simulink library "state_manager_lib"  (R2016b)
settings: Solver=ode45  StartTime=0.0  StopTime=10.0  RelTol=1e-3  EnableMultiTasking=on
undefined symbols (not defined in the file): ase_imu_p_indx, ase_local_mode_docking, ase_local_mode_map, ase_local_mode_perching, ase_ml_p_indx, ase_of_num_aug, ase_of_p_indx, ase_total_num_states, aug_state_enum, ml_omega_aug, ml_P_cam_ISS_ISS, ml_quat_ISS2cam, ml_vel_aug, of_omega_aug, of_vel_aug, tun_abp_p_dockcam_imu_est, tun_abp_p_navcam_imu_est, tun_abp_p_perchcam_imu_est, tun_abp_q_body2dockcam, tun_abp_q_body2navcam, tun_abp_q_body2perchcam, tun_ase_enable_of, tun_ase_ml_forward_projection_time
libraries: math_utils x8, simulink x7
settings Model: Creator=jfusco1  LastModifiedBy=jfusco1
settings DataIOCC: LimitDataPoints=on  SaveFormat=Array
settings OptimizationCC: LifeSpan=inf
settings DebuggingCC: AllowSymbolicDim=off  SFUnexpectedBacktrackingDiag=warning  SFNoUnconditionalDefaultTransitionDiag=warning  SFExecutionAtInitializationDiag=none
settings HardwareCC: ProdBitPerPointer=32  ProdBitPerSizeT=32  ProdBitPerPtrDiffT=32  ProdLargestAtomicFloat=None  ProdIntDivRoundTo=Undefined  ProdEndianess=Unspecified  ProdWordSize=32  ProdHWDeviceType=32-bit Generic
settings ModelReferenceCC: PropagateSignalLabelsOutOfModel=off
settings GRTTargetCC: TargetLangStandard=C89/C90 (ANSI)  GeneratePreprocessorConditionals=Disable all
settings ConfigComp: CovMetricSettings=dw  CovHtmlReporting=on  CovSaveCumulativeToWorkspaceVar=on  CovSaveSingleToWorkspaceVar=on  CovExternalEMLEnable=off

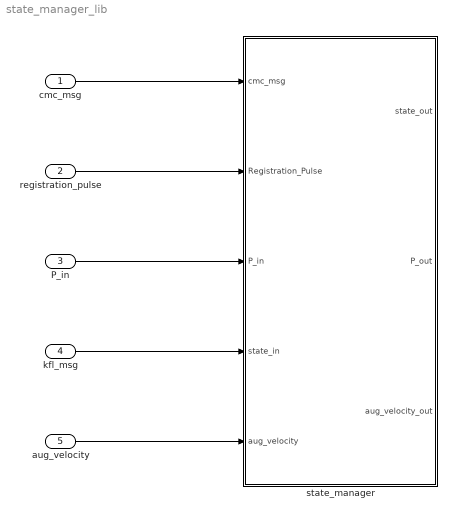
== system state_manager_lib ==
  cmc_msg : Inport  OutDataTypeStr=Bus: cmc_msg
  registration_pulse : Inport  Port=2  OutDataTypeStr=Bus: cvs_registration_pulse
  P_in : Inport  Port=3
  kfl_msg : Inport  Port=4  OutDataTypeStr=Bus: kfl_msg
  aug_velocity : Inport  Port=5
  state_manager : Subsystem
  wires:
  registration_pulse/1 -> state_manager/2(Registration_Pulse)
  kfl_msg/1 -> state_manager/4(state_in)
  P_in/1 -> state_manager/3(P_in)
  aug_velocity/1 -> state_manager/5(aug_velocity)
  cmc_msg/1 -> state_manager/1(cmc_msg)

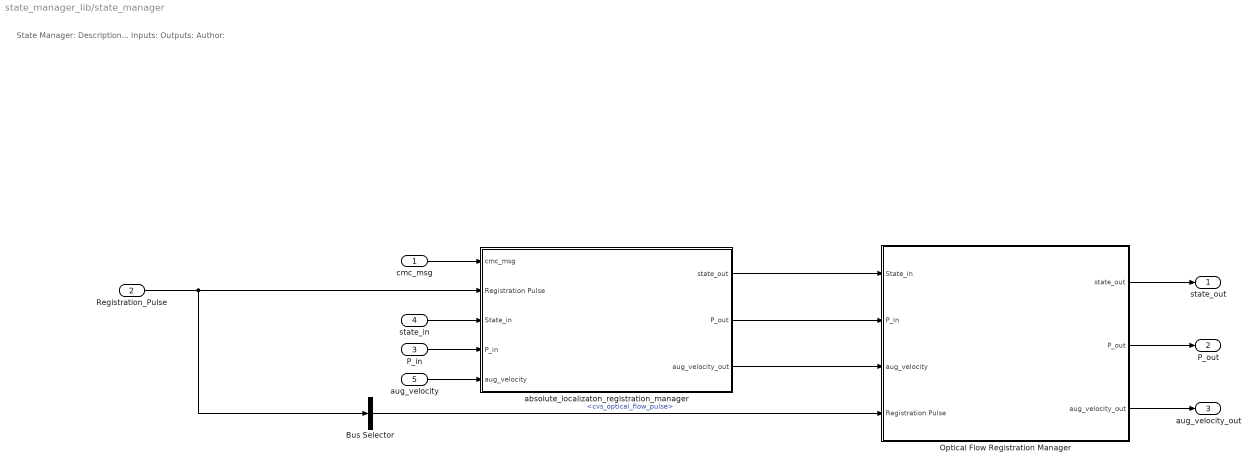
== system state_manager_lib/state_manager ==
  note: State Manager:
      | Description...
      |
      | Inputs:
      |
      | Outputs:
      |
      | Author:
  cmc_msg : Inport
  Registration_Pulse : Inport  Port=2
  P_in : Inport  Port=3  OutDataTypeStr=ase_cov_datatype
  state_in : Inport  Port=4
  aug_velocity : Inport  Port=5
  Bus Selector : BusSelector  OutputSignals=cvs_optical_flow_pulse
  Optical Flow Registration Manager : Subsystem
  absolute_localizaton_registration_manager : Subsystem
  state_out : Outport
  P_out : Outport  Port=2
  aug_velocity_out : Outport  Port=3
  wires:
  Optical Flow Registration Manager/3(aug_velocity_out) -> aug_velocity_out/1
  absolute_localizaton_registration_manager/3(aug_velocity_out) -> Optical Flow Registration Manager/3(aug_velocity)
  aug_velocity/1 -> absolute_localizaton_registration_manager/5(aug_velocity)
  state_in/1 -> absolute_localizaton_registration_manager/3(State_in)
  P_in/1 -> absolute_localizaton_registration_manager/4(P_in)
  absolute_localizaton_registration_manager/1(state_out) -> Optical Flow Registration Manager/1(State_in)
  Registration_Pulse/1 -> Bus Selector/1, absolute_localizaton_registration_manager/2(Registration Pulse)
  Bus Selector/1 -> Optical Flow Registration Manager/4(Registration Pulse)  "<cvs_optical_flow_pulse>"
  Optical Flow Registration Manager/1(state_out) -> state_out/1
  Optical Flow Registration Manager/2(P_out) -> P_out/1
  absolute_localizaton_registration_manager/2(P_out) -> Optical Flow Registration Manager/2(P_in)
  cmc_msg/1 -> absolute_localizaton_registration_manager/1(cmc_msg)

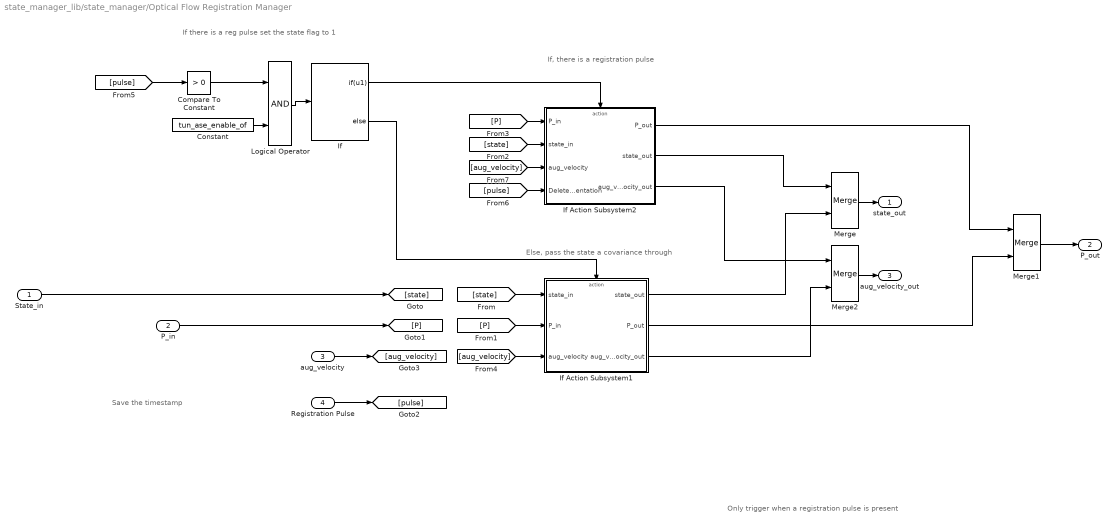
== system state_manager_lib/state_manager/Optical Flow Registration Manager ==
  note: Only trigger when a registration pulse is present
  note: If, there is a registration pulse
  note: Else, pass the state a covariance through
  note: Save the timestamp
  note: If there is a reg pulse set the state flag to 1
  State_in : Inport
  P_in : Inport  Port=2
  aug_velocity : Inport  Port=3
  Registration Pulse : Inport  Port=4
  Compare To Constant : simulink/Logic and Bit Operations/Compare To Constant  relop=>  const=0  OutDataTypeStr=boolean
  Constant : Constant  Value=tun_ase_enable_of
  If : If  IfExpression=u1
  If Action Subsystem1 : Subsystem  TreatAsAtomicUnit=on
  If Action Subsystem2 : Subsystem  TreatAsAtomicUnit=on
  Logical Operator : Logic  AllPortsSameDT=off  OutDataTypeStr=boolean
  Merge : Merge
  Merge1 : Merge
  Merge2 : Merge
  state_out : Outport
  P_out : Outport  Port=2
  aug_velocity_out : Outport  Port=3
  wires:
  If Action Subsystem1/3(aug_velocity_out) -> Merge2/2
  If Action Subsystem2/3(aug_velocity_out) -> Merge2/1
  Merge2/1 -> aug_velocity_out/1
  [aug_velocity] -> If Action Subsystem1/3(aug_velocity)
  [aug_velocity] -> If Action Subsystem2/3(aug_velocity)
  aug_velocity/1 -> [aug_velocity]
  [state] -> If Action Subsystem1/1(state_in)
  P_in/1 -> [P]
  [P] -> If Action Subsystem1/2(P_in)
  If/2 -> If Action Subsystem1/Action
  If/1 -> If Action Subsystem2/Action
  If Action Subsystem2/2(state_out) -> Merge/1
  [state] -> If Action Subsystem2/2(state_in)
  [P] -> If Action Subsystem2/1(P_in)
  If Action Subsystem2/1(P_out) -> Merge1/1
  Merge/1 -> state_out/1
  Merge1/1 -> P_out/1
  Logical Operator/1 -> If/1
  Compare To Constant/1 -> Logical Operator/1
  Constant/1 -> Logical Operator/2
  If Action Subsystem1/1(state_out) -> Merge/2
  If Action Subsystem1/2(P_out) -> Merge1/2
  State_in/1 -> [state]
  Registration Pulse/1 -> [pulse]
  [pulse] -> Compare To Constant/1
  [pulse] -> If Action Subsystem2/4(Deleted Augmentation)

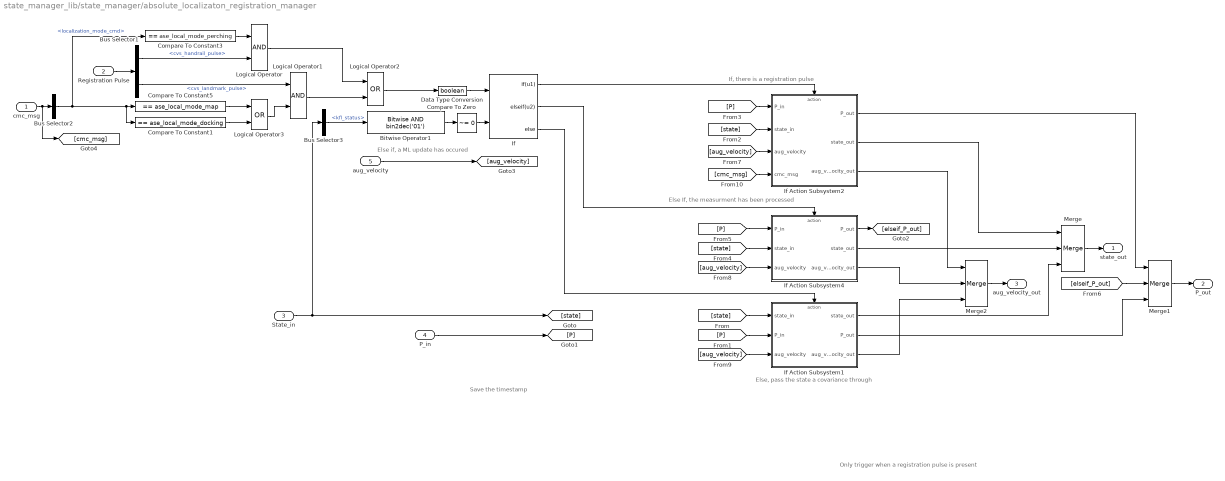
== system state_manager_lib/state_manager/absolute_localizaton_registration_manager ==
  note: Else If, the measurment has been processed
  note: Save the timestamp
  note: Else, pass the state a covariance through
  note: If, there is a registration pulse
  note: Only trigger when a registration pulse is present
  note: Else if, a ML update has occured
  cmc_msg : Inport
  Registration Pulse : Inport  Port=2
  State_in : Inport  Port=3
  P_in : Inport  Port=4
  aug_velocity : Inport  Port=5
  Bitwise Operator1 : simulink/Logic and Bit Operations/Bitwise Operator  logicop=AND  UseBitMask=on  BitMask=bin2dec('01')  BitMaskRealWorld=Stored Integer
  Bus Selector1 : BusSelector  OutputSignals=cvs_handrail_pulse,cvs_landmark_pulse
  Bus Selector2 : BusSelector  OutputSignals=localization_mode_cmd
  Bus Selector3 : BusSelector  OutputSignals=kfl_status
  Compare To Constant1 : simulink/Logic and Bit Operations/Compare To Constant  relop===  const=ase_local_mode_docking  OutDataTypeStr=boolean
  Compare To Constant3 : simulink/Logic and Bit Operations/Compare To Constant  relop===  const=ase_local_mode_perching  OutDataTypeStr=boolean
  Compare To Constant5 : simulink/Logic and Bit Operations/Compare To Constant  relop===  const=ase_local_mode_map  OutDataTypeStr=boolean
  Compare To Zero : simulink/Logic and Bit Operations/Compare To Zero  relop=~=  OutDataTypeStr=boolean
  Data Type Conversion : DataTypeConversion  OutDataTypeStr=boolean
  If : If  NumInputs=2  IfExpression=u1  ElseIfExpressions=u2
  If Action Subsystem1 : Subsystem  TreatAsAtomicUnit=on
  If Action Subsystem2 : Subsystem  TreatAsAtomicUnit=on
  If Action Subsystem4 : Subsystem  TreatAsAtomicUnit=on
  Logical Operator : Logic  AllPortsSameDT=off  OutDataTypeStr=boolean
  Logical Operator1 : Logic  AllPortsSameDT=off  OutDataTypeStr=boolean
  Logical Operator2 : Logic  Operator=OR  AllPortsSameDT=off  OutDataTypeStr=boolean
  Logical Operator3 : Logic  Operator=OR  AllPortsSameDT=off  OutDataTypeStr=boolean
  Merge : Merge  Inputs=3
  Merge1 : Merge  Inputs=3
  Merge2 : Merge  Inputs=3
  state_out : Outport
  P_out : Outport  Port=2
  aug_velocity_out : Outport  Port=3
  wires:
  If Action Subsystem1/3(aug_velocity_out) -> Merge2/3
  If Action Subsystem4/3(aug_velocity_out) -> Merge2/2
  If Action Subsystem2/3(aug_velocity_out) -> Merge2/1
  Merge2/1 -> aug_velocity_out/1
  [aug_velocity] -> If Action Subsystem1/3(aug_velocity)
  [aug_velocity] -> If Action Subsystem4/3(aug_velocity)
  [aug_velocity] -> If Action Subsystem2/3(aug_velocity)
  aug_velocity/1 -> [aug_velocity]
  Merge1/1 -> P_out/1
  [P] -> If Action Subsystem4/1(P_in)
  [state] -> If Action Subsystem4/2(state_in)
  Merge/1 -> state_out/1
  If Action Subsystem2/1(P_out) -> Merge1/1
  [P] -> If Action Subsystem2/1(P_in)
  If/2 -> If Action Subsystem4/Action
  [state] -> If Action Subsystem2/2(state_in)
  If Action Subsystem2/2(state_out) -> Merge/1
  If/1 -> If Action Subsystem2/Action
  If/3 -> If Action Subsystem1/Action
  [P] -> If Action Subsystem1/2(P_in)
  P_in/1 -> [P]
  [state] -> If Action Subsystem1/1(state_in)
  If Action Subsystem1/2(P_out) -> Merge1/3
  [elseif_P_out] -> Merge1/2
  Data Type Conversion/1 -> If/1
  If Action Subsystem4/1(P_out) -> [elseif_P_out]
  If Action Subsystem1/1(state_out) -> Merge/3
  If Action Subsystem4/2(state_out) -> Merge/2
  State_in/1 -> [state], Bus Selector3/1
  Bus Selector3/1 -> Bitwise Operator1/1  "<kfl_status>"
  Compare To Zero/1 -> If/2
  Bitwise Operator1/1 -> Compare To Zero/1
  Bus Selector2/1 -> Compare To Constant3/1, Compare To Constant1/1, Compare To Constant5/1  "<localization_mode_cmd>"
  cmc_msg/1 -> [cmc_msg], Bus Selector2/1
  Registration Pulse/1 -> Bus Selector1/1
  Logical Operator2/1 -> Data Type Conversion/1
  Logical Operator1/1 -> Logical Operator2/2
  Logical Operator/1 -> Logical Operator2/1
  Bus Selector1/1 -> Logical Operator/2  "<cvs_handrail_pulse>"
  Bus Selector1/2 -> Logical Operator1/1  "<cvs_landmark_pulse>"
  Compare To Constant3/1 -> Logical Operator/1
  [cmc_msg] -> If Action Subsystem2/4(cmc_msg)
  Compare To Constant5/1 -> Logical Operator3/1
  Compare To Constant1/1 -> Logical Operator3/2
  Logical Operator3/1 -> Logical Operator1/2

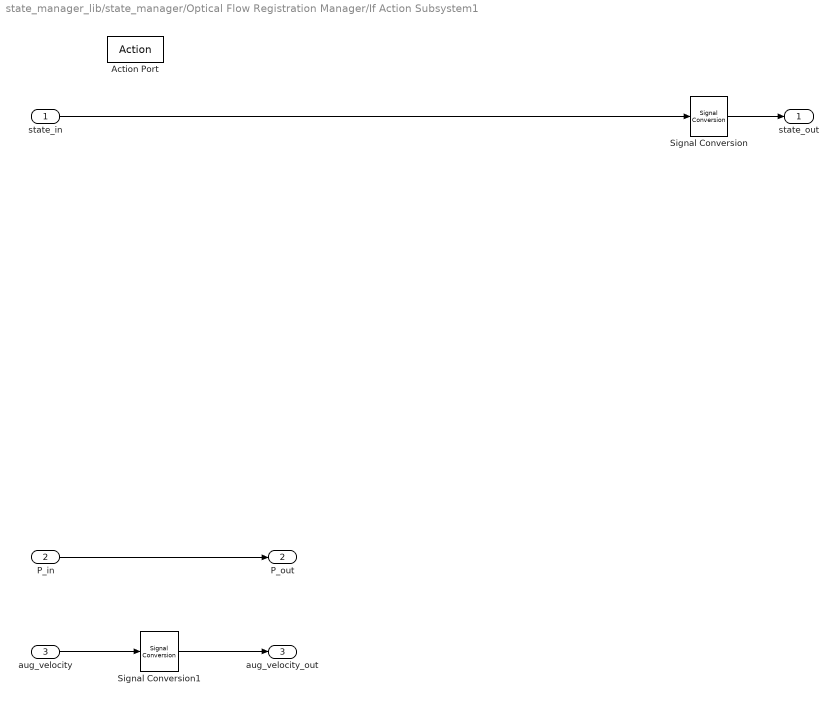
== system state_manager_lib/state_manager/Optical Flow Registration Manager/If Action Subsystem1 ==
  state_in : Inport
  P_in : Inport  Port=2
  aug_velocity : Inport  Port=3
  Action Port : ActionPort
  Signal Conversion : SignalConversion  OverrideOpt=off
  Signal Conversion1 : SignalConversion  OverrideOpt=off
  state_out : Outport
  P_out : Outport  Port=2
  aug_velocity_out : Outport  Port=3
  wires:
  Signal Conversion1/1 -> aug_velocity_out/1
  aug_velocity/1 -> Signal Conversion1/1
  P_in/1 -> P_out/1
  Signal Conversion/1 -> state_out/1
  state_in/1 -> Signal Conversion/1

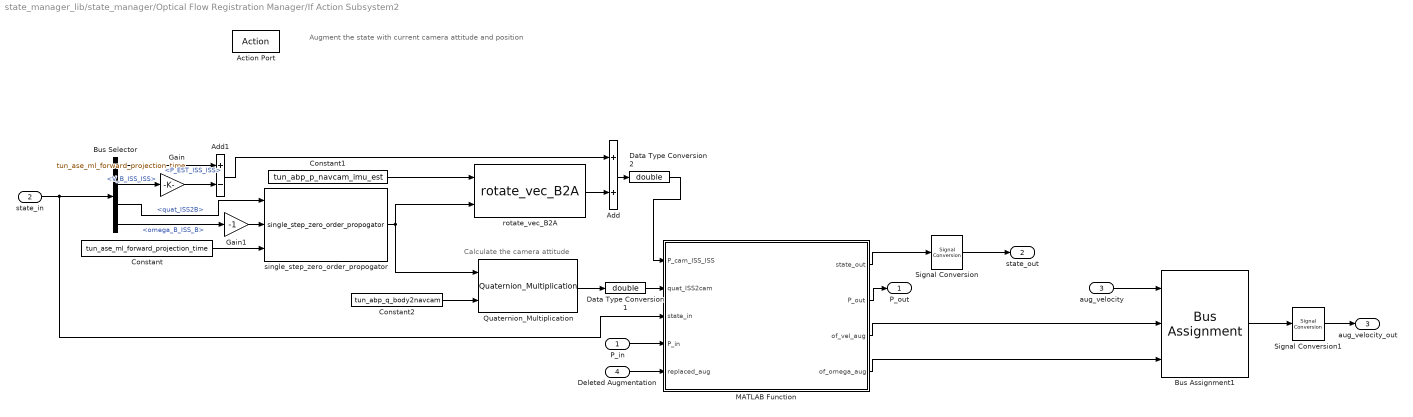
== system state_manager_lib/state_manager/Optical Flow Registration Manager/If Action Subsystem2 ==
  note: Augment the state with current camera attitude and position
  note: Calculate the camera attitude
  P_in : Inport
  state_in : Inport  Port=2
  aug_velocity : Inport  Port=3
  Deleted Augmentation : Inport  Port=4
  Action Port : ActionPort
  Add : Sum
  Add1 : Sum  Inputs=+-
  Bus Assignment1 : BusAssignment  AssignedSignals=of_vel_aug,of_omega_aug
  Bus Selector : BusSelector  OutputSignals=P_EST_ISS_ISS,V_B_ISS_ISS,quat_ISS2B,omega_B_ISS_B
  Constant : Constant  Value=tun_ase_ml_forward_projection_time
  Constant1 : Constant  Value=tun_abp_p_navcam_imu_est
  Constant2 : Constant  Value=tun_abp_q_body2navcam
  Data Type Conversion1 : DataTypeConversion  OutDataTypeStr=double
  Data Type Conversion2 : DataTypeConversion  OutDataTypeStr=double
  Gain : Gain  Gain=tun_ase_ml_forward_projection_time
  Gain1 : Gain  Gain=-1
  MATLAB Function : MATLAB Function  TreatAsAtomicUnit=on
  Quaternion_Multiplication : math_utils/Quaternion_Multiplication  SystemSampleTime=-1
  Signal Conversion : SignalConversion  OverrideOpt=off
  Signal Conversion1 : SignalConversion  OverrideOpt=off
  rotate_vec_B2A : math_utils/rotate_vec_B2A  SystemSampleTime=-1
  single_step_zero_order_propogator : math_utils/single_step_zero_order_propogator  SystemSampleTime=-1
  P_out : Outport
  state_out : Outport  Port=2
  aug_velocity_out : Outport  Port=3
  wires:
  Signal Conversion1/1 -> aug_velocity_out/1
  Bus Assignment1/1 -> Signal Conversion1/1
  MATLAB Function/4(of_omega_aug) -> Bus Assignment1/3
  MATLAB Function/3(of_vel_aug) -> Bus Assignment1/2
  aug_velocity/1 -> Bus Assignment1/1
  MATLAB Function/1(state_out) -> Signal Conversion/1
  state_in/1 -> MATLAB Function/3(state_in), Bus Selector/1
  Constant2/1 -> Quaternion_Multiplication/2
  Bus Selector/3 -> single_step_zero_order_propogator/1  "<quat_ISS2B>"
  Quaternion_Multiplication/1 -> Data Type Conversion1/1
  P_in/1 -> MATLAB Function/4(P_in)
  MATLAB Function/2(P_out) -> P_out/1
  Signal Conversion/1 -> state_out/1
  Bus Selector/4 -> Gain1/1  "<omega_B_ISS_B>"
  Gain1/1 -> single_step_zero_order_propogator/2
  Constant/1 -> single_step_zero_order_propogator/3
  Gain/1 -> Add1/2
  Add1/1 -> Add/1
  rotate_vec_B2A/1 -> Add/2
  Bus Selector/2 -> Gain/1  "<V_B_ISS_ISS>"
  Bus Selector/1 -> Add1/1  "<P_EST_ISS_ISS>"
  Constant1/1 -> rotate_vec_B2A/1
  Data Type Conversion1/1 -> MATLAB Function/2(quat_ISS2cam)
  Data Type Conversion2/1 -> MATLAB Function/1(P_cam_ISS_ISS)
  Add/1 -> Data Type Conversion2/1
  Deleted Augmentation/1 -> MATLAB Function/5(replaced_aug)
  single_step_zero_order_propogator/1 -> Quaternion_Multiplication/1, rotate_vec_B2A/2

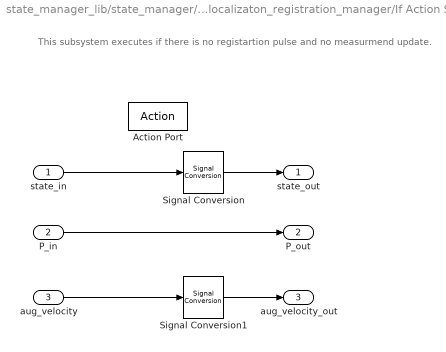
== system state_manager_lib/state_manager/absolute_localizaton_registration_manager/If Action Subsystem1 ==
  note: This subsystem executes if there is no registartion pulse and no measurmend update.
  state_in : Inport
  P_in : Inport  Port=2
  aug_velocity : Inport  Port=3
  Action Port : ActionPort
  Signal Conversion : SignalConversion  OverrideOpt=off
  Signal Conversion1 : SignalConversion  OverrideOpt=off
  state_out : Outport
  P_out : Outport  Port=2
  aug_velocity_out : Outport  Port=3
  wires:
  Signal Conversion1/1 -> aug_velocity_out/1
  aug_velocity/1 -> Signal Conversion1/1
  Signal Conversion/1 -> state_out/1
  P_in/1 -> P_out/1
  state_in/1 -> Signal Conversion/1

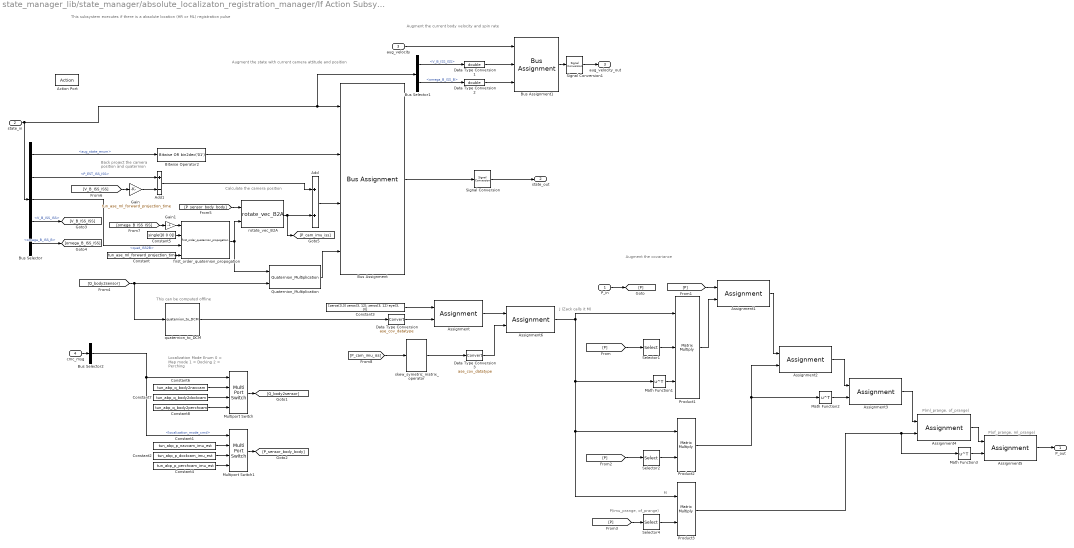
== system state_manager_lib/state_manager/absolute_localizaton_registration_manager/If Action Subsystem2 ==
  note: This subsystem executes if there is a absolute location (HR or ML) registration pulse
  note: Augment the covariance
  note: Augment the current body velocity and spin rate
  note: P(of_prange, ml_prange)
  note: P(ml_prange, of_prange)
  note: M
  note: P(imu_prange, of_prange)
  note: Augment the state with current camera attitude and position
  note: J (Zack calls it M)
  note: This can be computed offline
  note: Calculate the camera position
  note: Back project the camera position and quaternion
  note: Localization Mode Enum
      | 0 = Map mode
      | 1 = Docking
      | 2 = Perching
  P_in : Inport
  state_in : Inport  Port=2  OutDataTypeStr=Bus: kfl_msg
  aug_velocity : Inport  Port=3
  cmc_msg : Inport  Port=4
  Action Port : ActionPort
  Add : Sum
  Add1 : Sum  Inputs=+-
  Assignment : Assignment  NumberOfDimensions=2  DiagnosticForDimensions=Warning  IndexOptions=Index vector (dialog),Index vector (dialog)  Indices=[1:3],[1:3]  OutputSizes=1,1
  Assignment1 : Assignment  NumberOfDimensions=2  DiagnosticForDimensions=Warning  IndexOptions=Index vector (dialog),Index vector (dialog)  Indices=ase_ml_p_indx,ase_ml_p_indx  OutputSizes=1,1
      settings: AttributesFormatString=Indices:%<Indices>
  Assignment2 : Assignment  NumberOfDimensions=2  DiagnosticForDimensions=Warning  IndexOptions=Index vector (dialog),Index vector (dialog)  Indices=ase_ml_p_indx,ase_imu_p_indx  OutputSizes=1,1
      settings: AttributesFormatString=Indices:%<Indices>
  Assignment3 : Assignment  NumberOfDimensions=2  DiagnosticForDimensions=Warning  IndexOptions=Index vector (dialog),Index vector (dialog)  Indices=ase_imu_p_indx,ase_ml_p_indx  OutputSizes=1,1
      settings: AttributesFormatString=Indices:%<Indices>
  Assignment4 : Assignment  NumberOfDimensions=2  DiagnosticForDimensions=Warning  IndexOptions=Index vector (dialog),Index vector (dialog)  Indices=16:21,ase_of_p_indx  OutputSizes=1,1
      settings: AttributesFormatString=Indices:%<Indices>
  Assignment5 : Assignment  NumberOfDimensions=2  DiagnosticForDimensions=Warning  IndexOptions=Index vector (dialog),Index vector (dialog)  Indices=ase_of_p_indx,16:21  OutputSizes=1,1
      settings: AttributesFormatString=Indices:%<Indices>
  Assignment6 : Assignment  NumberOfDimensions=2  DiagnosticForDimensions=Warning  IndexOptions=Index vector (dialog),Index vector (dialog)  Indices=[4:6],[1:3]  OutputSizes=1,1
  Bitwise Operator2 : simulink/Logic and Bit Operations/Bitwise Operator  logicop=OR  UseBitMask=on  BitMask=bin2dec('01')  BitMaskRealWorld=Stored Integer
  Bus Assignment : BusAssignment  AssignedSignals=aug_state_enum,ml_P_cam_ISS_ISS,ml_quat_ISS2cam
  Bus Assignment1 : BusAssignment  AssignedSignals=ml_vel_aug,ml_omega_aug
  Bus Selector : BusSelector  OutputSignals=aug_state_enum,P_EST_ISS_ISS,quat_ISS2B,V_B_ISS_ISS,omega_B_ISS_B
  Bus Selector1 : BusSelector  OutputSignals=V_B_ISS_ISS,omega_B_ISS_B
  Bus Selector2 : BusSelector  OutputSignals=localization_mode_cmd
  Constant : Constant  Value=tun_ase_ml_forward_projection_time
  Constant1 : Constant  Value=tun_abp_p_navcam_imu_est
  Constant2 : Constant  Value=tun_abp_p_dockcam_imu_est
  Constant3 : Constant  Value=[zeros(3,3) zeros(3, 12); zeros(3, 12) eye(3, 3)]  OutDataTypeStr=ase_cov_datatype
  Constant4 : Constant  Value=tun_abp_p_perchcam_imu_est
  Constant5 : Constant  Value=single([0 0 0])
  Constant6 : Constant  Value=tun_abp_q_body2navcam
  Constant7 : Constant  Value=tun_abp_q_body2dockcam
  Constant8 : Constant  Value=tun_abp_q_body2perchcam
  Data Type Conversion : DataTypeConversion  OutDataTypeStr=ase_cov_datatype
  Data Type Conversion1 : DataTypeConversion  OutDataTypeStr=double
  Data Type Conversion2 : DataTypeConversion  OutDataTypeStr=double
  Data Type Conversion3 : DataTypeConversion  OutDataTypeStr=ase_cov_datatype
  Gain : Gain  Gain=tun_ase_ml_forward_projection_time
  Gain1 : Gain  Gain=-1
  Math Function1 : Math  Operator=transpose  SaturateOnIntegerOverflow=on
  Math Function2 : Math  Operator=transpose  SaturateOnIntegerOverflow=on
  Math Function3 : Math  Operator=transpose  SaturateOnIntegerOverflow=on
  Multiport Switch : MultiPortSwitch  DataPortOrder=Zero-based contiguous
  Multiport Switch1 : MultiPortSwitch  DataPortOrder=Zero-based contiguous
  Product1 : Product  Inputs=3  Multiplication=Matrix(*)
  Product2 : Product  Multiplication=Matrix(*)
  Product3 : Product  Multiplication=Matrix(*)
  Quaternion_Multiplication : math_utils/Quaternion_Multiplication  SystemSampleTime=-1
  Selector1 : Selector  NumberOfDimensions=2  InputPortWidth=3  IndexOptions=Index vector (dialog),Index vector (dialog)  Indices=[1:15],[1:15]  OutputSizes=1,1
  Selector2 : Selector  NumberOfDimensions=2  InputPortWidth=3  IndexOptions=Index vector (dialog),Index vector (dialog)  Indices=[1:15],[1:15]  OutputSizes=1,1
      settings: AttributesFormatString=Indices:%<Indices>
  Selector4 : Selector  NumberOfDimensions=2  InputPortWidth=3  IndexOptions=Index vector (dialog),Index vector (dialog)  Indices=[1:15],ase_of_p_indx  OutputSizes=1,1
      settings: AttributesFormatString=Indices: %<Indices>
  Signal Conversion : SignalConversion  OverrideOpt=off
  Signal Conversion1 : SignalConversion  OverrideOpt=off
  first_order_quaternion_propogation : math_utils/first_order_quaternion_propogation  SystemSampleTime=-1
  quaternion_to_DCM : math_utils/quaternion_to_DCM  SystemSampleTime=-1
  rotate_vec_B2A : math_utils/rotate_vec_B2A  SystemSampleTime=-1
  skew_symetric_matrix_operator : math_utils/skew_symetric_matrix_operator  SystemSampleTime=-1
  P_out : Outport
  state_out : Outport  Port=2
  aug_velocity_out : Outport  Port=3
  wires:
  Signal Conversion1/1 -> aug_velocity_out/1
  Data Type Conversion2/1 -> Bus Assignment1/3
  Data Type Conversion1/1 -> Bus Assignment1/2
  Bus Selector1/2 -> Data Type Conversion2/1  "<omega_B_ISS_B>"
  Bus Selector1/1 -> Data Type Conversion1/1  "<V_B_ISS_ISS>"
  Bus Assignment1/1 -> Signal Conversion1/1
  aug_velocity/1 -> Bus Assignment1/1
  Assignment5/1 -> P_out/1
  Assignment4/1 -> Assignment5/1
  Product3/1 -> Assignment4/2, Math Function3/1
  Math Function3/1 -> Assignment5/2
  Assignment3/1 -> Assignment4/1
  Selector4/1 -> Product3/2
  [P] -> Selector4/1
  Signal Conversion/1 -> state_out/1
  Assignment6/1 -> Product1/1, Math Function1/1, Product2/1, Product3/1
  P_in/1 -> [P]
  quaternion_to_DCM/1 -> Data Type Conversion/1
  Constant3/1 -> Assignment/1
  [Q_body2sensor] -> quaternion_to_DCM/1, Quaternion_Multiplication/2
  Bitwise Operator2/1 -> Bus Assignment/2
  state_in/1 -> Bus Assignment/1, Bus Selector1/1, Bus Selector/1
  Bus Assignment/1 -> Signal Conversion/1
  [P_sensor_body_body] -> rotate_vec_B2A/1
  Math Function1/1 -> Product1/3
  Selector1/1 -> Product1/2
  [P] -> Selector1/1
  [P] -> Assignment1/1
  Product1/1 -> Assignment1/2
  [P] -> Selector2/1
  Selector2/1 -> Product2/2
  Assignment1/1 -> Assignment2/1
  Assignment2/1 -> Assignment3/1
  Product2/1 -> Assignment2/2, Math Function2/1
  Math Function2/1 -> Assignment3/2
  Bus Selector/1 -> Bitwise Operator2/1  "<aug_state_enum>"
  Data Type Conversion/1 -> Assignment/2
  cmc_msg/1 -> Bus Selector2/1
  Multiport Switch/1 -> [Q_body2sensor]
  Multiport Switch1/1 -> [P_sensor_body_body]
  Bus Selector/4 -> [V_B_ISS_ISS]  "<V_B_ISS_ISS>"
  Bus Selector/5 -> [omega_B_ISS_ISS]  "<omega_B_ISS_B>"
  [V_B_ISS_ISS] -> Gain/1
  Gain/1 -> Add1/2
  [omega_B_ISS_ISS] -> Gain1/1
  Gain1/1 -> first_order_quaternion_propogation/1
  Constant/1 -> first_order_quaternion_propogation/4
  Add/1 -> Bus Assignment/3
  Bus Selector/2 -> Add1/1  "<P_EST_ISS_ISS>"
  Add1/1 -> Add/1
  Bus Selector/3 -> first_order_quaternion_propogation/3  "<quat_ISS2B>"
  first_order_quaternion_propogation/1 -> rotate_vec_B2A/2, Quaternion_Multiplication/1
  Quaternion_Multiplication/1 -> Bus Assignment/4
  Bus Selector2/1 -> Multiport Switch1/1, Multiport Switch/1  "<localization_mode_cmd>"
  Constant6/1 -> Multiport Switch/2
  Constant7/1 -> Multiport Switch/3
  Constant8/1 -> Multiport Switch/4
  Constant1/1 -> Multiport Switch1/2
  Constant2/1 -> Multiport Switch1/3
  Constant4/1 -> Multiport Switch1/4
  rotate_vec_B2A/1 -> [P_cam_imu_iss], Add/2
  [P_cam_imu_iss] -> skew_symetric_matrix_operator/1
  Assignment/1 -> Assignment6/1
  skew_symetric_matrix_operator/1 -> Data Type Conversion3/1
  Data Type Conversion3/1 -> Assignment6/2
  Constant5/1 -> first_order_quaternion_propogation/2

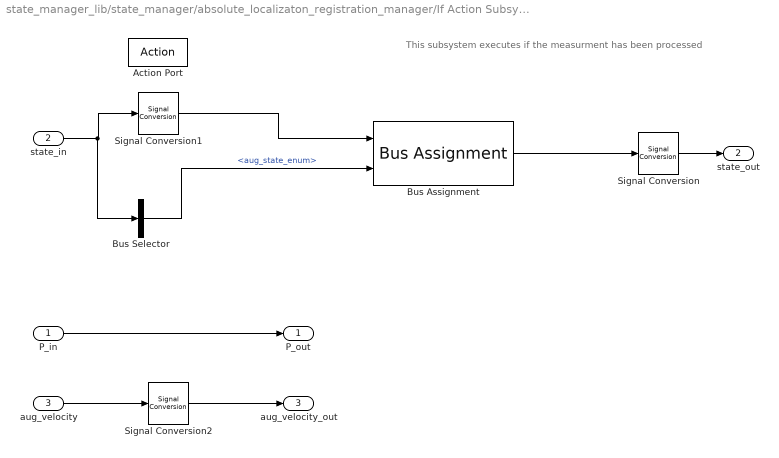
== system state_manager_lib/state_manager/absolute_localizaton_registration_manager/If Action Subsystem4 ==
  note: This subsystem executes if the measurment has been processed
  P_in : Inport
  state_in : Inport  Port=2
  aug_velocity : Inport  Port=3
  Action Port : ActionPort
  Bus Assignment : BusAssignment  AssignedSignals=aug_state_enum
  Bus Selector : BusSelector  OutputSignals=aug_state_enum
  Signal Conversion : SignalConversion  OverrideOpt=off
  Signal Conversion1 : SignalConversion  OverrideOpt=off
  Signal Conversion2 : SignalConversion  OverrideOpt=off
  P_out : Outport
  state_out : Outport  Port=2
  aug_velocity_out : Outport  Port=3
  wires:
  Signal Conversion2/1 -> aug_velocity_out/1
  aug_velocity/1 -> Signal Conversion2/1
  Bus Selector/1 -> Bus Assignment/2  "<aug_state_enum>"
  P_in/1 -> P_out/1
  state_in/1 -> Signal Conversion1/1, Bus Selector/1
  Bus Assignment/1 -> Signal Conversion/1
  Signal Conversion/1 -> state_out/1
  Signal Conversion1/1 -> Bus Assignment/1

== matlab function state_manager_lib/state_manager/Optical Flow Registration Manager/If Action Subsystem2/MATLAB Function ==
  data: P_cam_ISS_ISS input; quat_ISS2cam input; state_in input; state_out output Bus: kfl_msg; P_in input; P_out output size=[ase_total_num_states ase_total_num_states]; tun_abp_q_body2navcam parameter; tun_abp_p_navcam_imu_est parameter; ase_total_num_states parameter; ase_of_num_aug parameter; of_vel_aug output double; of_omega_aug output double; replaced_aug input
% From Zack's matlab filter.  This function add loads up the most recent
% camera attitude and position, as well as setting the aug_state_byte
function [state_out, P_out, of_vel_aug, of_omega_aug]   = augment_camera_of(P_cam_ISS_ISS, quat_ISS2cam, state_in, P_in, tun_abp_q_body2navcam, tun_abp_p_navcam_imu_est, ase_total_num_states, ase_of_num_aug, replaced_aug)
%#codegen
  [state_out, P_out, of_vel_aug, of_omega_aug] = eml_augment_camera_of(P_cam_ISS_ISS, quat_ISS2cam, state_in, P_in, tun_abp_q_body2navcam, tun_abp_p_navcam_imu_est, ase_total_num_states, ase_of_num_aug, replaced_aug);
end
